simulink model "ml_ss"  (R2019b)
settings: Solver=VariableStepAuto  StartTime=0.0  StopTime=30  RelTol=1e-3
values from neighbouring files (symbols this model uses):
  phi = 0.3    [adapt_scaling_factors.mat]    (also in scaling.m = max(input(:,2)); scaling_factors.mat)
  phi_dot = 4.08329955968    [adapt_scaling_factors.mat]    (also in scaling.m = max(input(:,4)); scaling_factors.mat = 2.60882756641)
  x = 5.94515732007    [adapt_scaling_factors.mat]    (also in myNeuralNetworkFunction.m = bsxfun(@plus,x,settings.xoffset); scaling.m = max(input(:,1)); scaling_factors.mat = 5.30104950894)
  x_dot = 1.32188519006    [adapt_scaling_factors.mat]    (also in scaling.m = max(input(:,3)); scaling_factors.mat = 1.12108693589)
libraries: simulink x2
settings Model: NumberOfSteps=10  Creator=Andrew  LastModifiedBy=Andrew

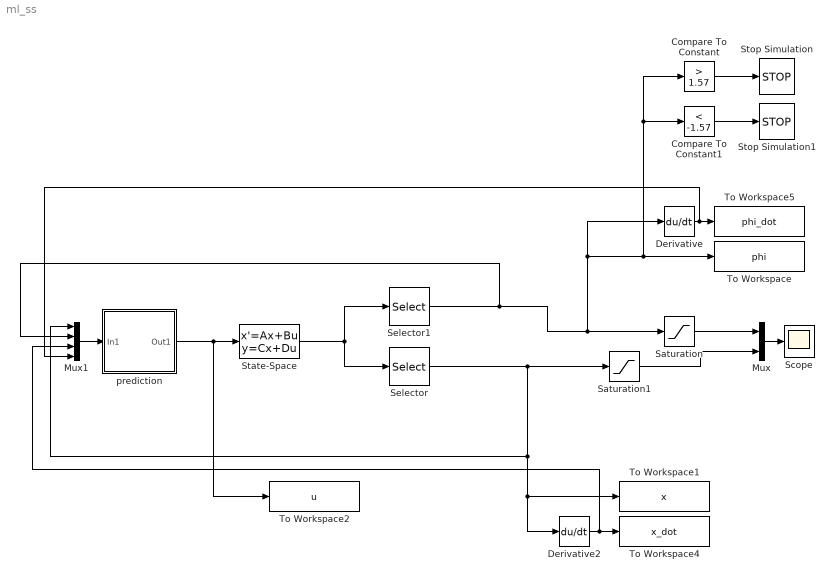
== system ml_ss ==
  Compare To Constant : simulink/Logic and Bit Operations/Compare To Constant  relop=>  const=1.57  OutDataTypeStr=boolean
  Compare To Constant1 : simulink/Logic and Bit Operations/Compare To Constant  relop=<  const=-1.57  OutDataTypeStr=boolean
  Derivative : Derivative
  Derivative2 : Derivative
  Mux : Mux  Inputs=2
  Mux1 : Mux
  Saturation : Saturate  UpperLimit=20  LowerLimit=-20
  Saturation1 : Saturate  UpperLimit=10000000  LowerLimit=-10000000
  Scope : Scope
  Selector : Selector  InputPortWidth=2  IndexOptions=Index vector (dialog)  Indices=[1]  OutputSizes=1
  Selector1 : Selector  InputPortWidth=2  IndexOptions=Index vector (dialog)  Indices=[2]  OutputSizes=1
  State-Space : StateSpace  A=[0 1 0 0;0 -0.1818 2.6727 0;0 0 0 1;0 -0.4545 31.1818 0]  B=[0;1.8182;0;4.5455]  C=[1 0 0 0;0 0 1 0]  D=[0;0]  InitialCondition=[0 0 0 0]
  Stop Simulation : Stop
  Stop Simulation1 : Stop
  To Workspace : ToWorkspace  VariableName=phi  SampleTime=-1
  To Workspace1 : ToWorkspace  VariableName=x  SampleTime=-1
  To Workspace2 : ToWorkspace  VariableName=u  SampleTime=-1
  To Workspace4 : ToWorkspace  VariableName=x_dot  SampleTime=-1
  To Workspace5 : ToWorkspace  VariableName=phi_dot  SampleTime=-1
  "prediction " : Subsystem
  wires:
  Mux/1 -> Scope/1
  Saturation/1 -> Mux/1
  Saturation1/1 -> Mux/2
  State-Space/1 -> Selector1/1, Selector/1
  Selector/1 -> Mux1/1, To Workspace1/1, Derivative2/1, Saturation1/1
  Selector1/1 -> Mux1/2, Compare To Constant1/1, Compare To Constant/1, To Workspace/1, Derivative/1, Saturation/1
  Derivative/1 -> Mux1/4, To Workspace5/1
  Derivative2/1 -> Mux1/3, To Workspace4/1
  Compare To Constant1/1 -> Stop Simulation1/1
  Compare To Constant/1 -> Stop Simulation/1
  "prediction "/1(Out1) -> To Workspace2/1, State-Space/1
  Mux1/1 -> "prediction "/1(In1)

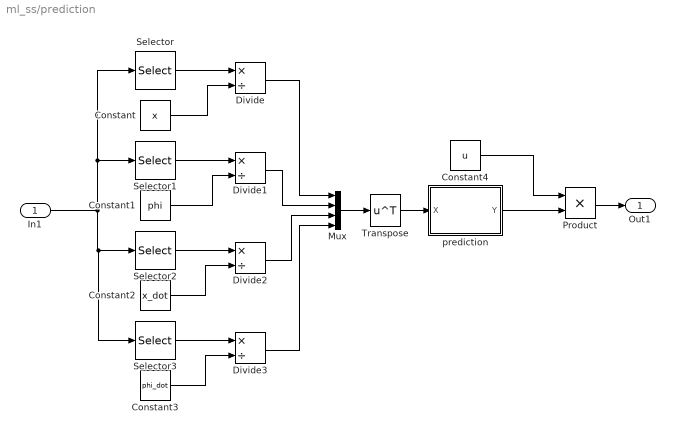
== system ml_ss/prediction  ==
  In1 : Inport
  Constant : Constant  Value=x
  Constant1 : Constant  Value=phi
  Constant2 : Constant  Value=x_dot
  Constant3 : Constant  Value=phi_dot
  Constant4 : Constant  Value=u
  Divide{,1..3} (4 alike) : Product  Inputs=*/
  Mux : Mux
  Product : Product
  Selector : Selector  InputPortWidth=4  IndexOptions=Index vector (dialog)  Indices=[1]  OutputSizes=1
  Selector1 : Selector  InputPortWidth=4  IndexOptions=Index vector (dialog)  Indices=[2]  OutputSizes=1
  Selector2 : Selector  InputPortWidth=4  IndexOptions=Index vector (dialog)  Indices=[3]  OutputSizes=1
  Selector3 : Selector  InputPortWidth=4  IndexOptions=Index vector (dialog)  Indices=[4]  OutputSizes=1
  Transpose : Math  Operator=transpose  SignedPower=off  SaturateOnIntegerOverflow=on
  "prediction " : MATLAB Function  TreatAsAtomicUnit=on
  Out1 : Outport
  wires:
  In1/1 -> Selector3/1, Selector2/1, Selector1/1, Selector/1
  Selector2/1 -> Divide2/1
  Selector3/1 -> Divide3/1
  Constant2/1 -> Divide2/2
  Constant3/1 -> Divide3/2
  Divide/1 -> Mux/1
  Divide1/1 -> Mux/2
  Divide2/1 -> Mux/3
  Divide3/1 -> Mux/4
  Mux/1 -> Transpose/1
  Transpose/1 -> "prediction "/1(X)
  Selector/1 -> Divide/1
  Constant/1 -> Divide/2
  Constant1/1 -> Divide1/2
  Selector1/1 -> Divide1/1
  "prediction "/1(Y) -> Product/2
  Product/1 -> Out1/1
  Constant4/1 -> Product/1

== matlab function ml_ss/prediction /prediction  ==
  data: X input; Y output
function Y = prediction(X) %#codegen
Mdl = loadLearnerForCoder('model');
Y = predict(Mdl,X);
end
